simulink model "PneumaticsSystem"  (R2019b)
settings: configuration reference "ConfigSet_PneumaticsSystem_Reference" (kept outside this file)
PostLoadFcn:
  | set_up_test_model()
model workspace (MAT data in the model file):
  PAtm = 101300
  Prm_PneumaticsSystem : Simulink.Parameter (value not decoded)
  SampleTime = 0.01
symbols that are objects in the model workspace (value not decoded): Prm_PneumaticsSystem
undefined symbols (not defined in the file): AirSuspensionBogie1Deflated, AirSuspensionPressure, AirSuspensionPressureSwitch, AirSuspPressureDiff, AuxiliaryReservoirPressure, AuxiliaryReservoirPressureSwitch, BECU1BrakeNotApplied, BECU1BrakeNotReleased, BECU1CarLoadPressureLow, BECU1EmergencyBrakeFailure, BECU1LoadPressureLow, BECU1ServiceBrakeFailure, BECU2CarLoadPressureLow, BECU2EmergencyBrakeFailure, BECULowRPressure, Bogie, BrakeCylinderControlPressure, BrakeCylinderPressure, BrakeCylinderPressureGauge, BrakeCylinderPressureSwitch, BrakeReservoirPressure, BrakeReservoirPressureSwitch, HornHighPressureSwitch, HornLowPressureSwitch, MainReservoirPipePressure, MainReservoirPipePressureSwitch, MainReservoirPressure, MainReservoirPressureGauge, MainReservoirPressureSwitch, MaxAxles, MRPS_TractionCutout, ORDPressureSwitch, PantographCylinderPressure, ParkBrakePressure, ParkBrakePressureGauge, ParkBrakePressureSwitch, PS2, PS3, SandingSystemPressure, SandingSystemPressureSwitch, SRPressureGauge, VCBCylinderPressure, VCBPressureSwitch
libraries: PneumaticLib x56, simulink x50, LatchesLib x7, FiltersLib x4, TimersLib x3, MathOperationsLib x3, VectorOperationsLib x1, simulink_extras x1
(part 3 of 3)

== system PneumaticsSystem/PneumaticsPerVehicle/PneumaticsSystem/MainReservoirSystem/MainReservoirPipe/FlowCalc ==
  MRPSelf : Inport
  MRPUpPressure : Inport  Port=2
  MRPDownPressure : Inport  Port=3
  MRPUpConnection : Inport  Port=4
  MRPDownConnection : Inport  Port=5
  MRPToBRFlowRate : Inport  Port=6
  MRPToAirSuspFlowRate : Inport  Port=7
  MRPToAuxRFlowRate : Inport  Port=8
  MRPToMRFlowRate : Inport  Port=9
  Add : Sum  Inputs=------
  Logical Operator : Logic  Operator=NOT  AllPortsSameDT=off  OutDataTypeStr=boolean
  Logical Operator1 : Logic  Operator=NOT  AllPortsSameDT=off  OutDataTypeStr=boolean
  MRP to Downstream Connection : PneumaticLib/SS Two Way Valve  d=0.01475  p_deadband=200
      settings: SourceProductName=Pneumatic
  MRP to Upstream Connection : PneumaticLib/SS Two Way Valve  d=0.01475  p_deadband=200
      settings: SourceProductName=Pneumatic
  Terminator1 : Terminator
  Terminator2 : Terminator
  Flow : Outport  VectorParamsAs1DForOutWhenUnconnected=off
  wires:
  Add/1 -> Flow/1  "flowMRP"
  MRPDownPressure/1 -> MRP to Downstream Connection/2
  MRPDownConnection/1 -> Logical Operator1/1
  MRPUpConnection/1 -> Logical Operator/1
  MRPUpPressure/1 -> MRP to Upstream Connection/2
  MRP to Upstream Connection/2 -> Terminator2/1
  Logical Operator/1 -> MRP to Upstream Connection/3
  MRPSelf/1 -> MRP to Downstream Connection/1, MRP to Upstream Connection/1
  MRP to Upstream Connection/1 -> Add/1  "MRPUpPressureFlowRate"
  MRP to Downstream Connection/1 -> Add/2  "MRPDownPressureFlowRate"
  MRP to Downstream Connection/2 -> Terminator1/1
  Logical Operator1/1 -> MRP to Downstream Connection/3
  MRPToMRFlowRate/1 -> Add/4  "MRPToMRFlowRate"
  MRPToAirSuspFlowRate/1 -> Add/5  "MRPToAirSuspFlowRate"
  MRPToBRFlowRate/1 -> Add/3  "MRPToBRFlowRate"
  MRPToAuxRFlowRate/1 -> Add/6  "MRPToMRFlowRate"

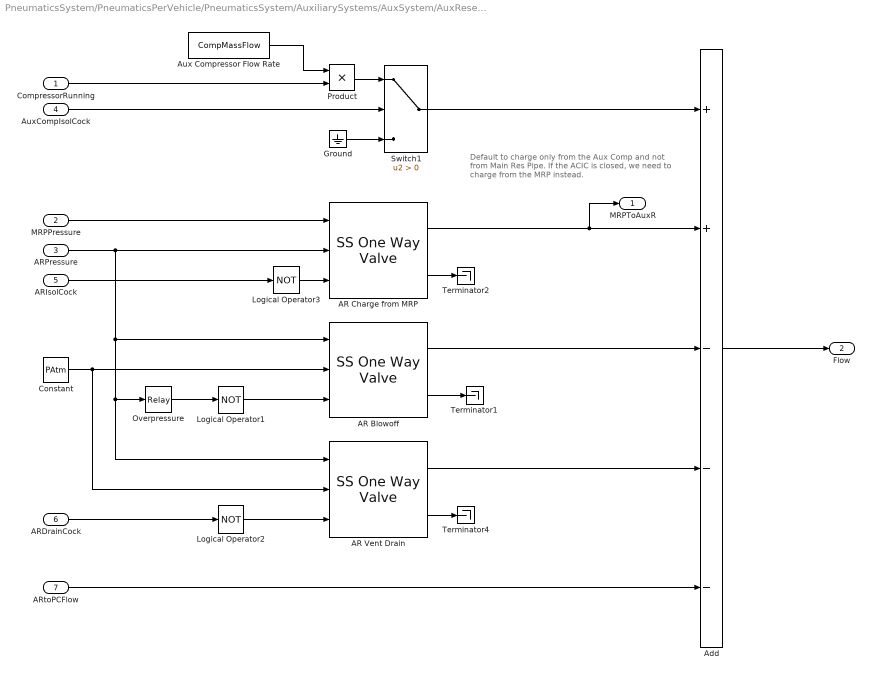
== system PneumaticsSystem/PneumaticsPerVehicle/PneumaticsSystem/AuxiliarySystems/AuxSystem/AuxReservoir/FlowCalc ==
  note: Default to charge only from the Aux Comp and not
      | from Main Res Pipe.
      | If the ACIC is closed, we need to charge from the
      | MRP instead.
  CompressorRunning : Inport
  MRPPressure : Inport  Port=2
  ARPressure : Inport  Port=3
  AuxCompIsolCock : Inport  Port=4
  ARIsolCock : Inport  Port=5
  ARDrainCock : Inport  Port=6
  ARtoPCFlow : Inport  Port=7
  AR Blowoff : PneumaticLib/SS One Way Valve  d=0.001  p_deadband=1000
      settings: SourceProductName=Train Library
  AR Charge from MRP : PneumaticLib/SS One Way Valve  d=0.0025  p_deadband=1000
      settings: SourceProductName=Train Library
  AR Vent Drain : PneumaticLib/SS One Way Valve  d=0.005  p_deadband=1000
      settings: SourceProductName=Train Library
  Add : Sum  Inputs=++---
  Aux Compressor Flow Rate : Constant  Value=CompMassFlow
  Constant : Constant  Value=PAtm
  Ground : Ground
  Logical Operator1 : Logic  Operator=NOT  AllPortsSameDT=off  OutDataTypeStr=boolean
  Logical Operator2 : Logic  Operator=NOT  AllPortsSameDT=off  OutDataTypeStr=boolean
  Logical Operator3 : Logic  Operator=NOT  AllPortsSameDT=off  OutDataTypeStr=boolean
  Overpressure : Relay  OnSwitchValue=BlowOffON + PAtm  OffSwitchValue=BlowOffOFF + PAtm
  Product : Product
  Switch1 : Switch  Criteria=u2 > Threshold
  Terminator1 : Terminator
  Terminator2 : Terminator
  Terminator4 : Terminator
  MRPToAuxR : Outport
  Flow : Outport  Port=2
  wires:
  Logical Operator2/1 -> AR Vent Drain/3
  AR Vent Drain/2 -> Terminator4/1
  Constant/1 -> AR Blowoff/2, AR Vent Drain/2
  AR Blowoff/2 -> Terminator1/1
  Add/1 -> Flow/1
  ARPressure/1 -> AR Vent Drain/1, Overpressure/1, AR Blowoff/1, AR Charge from MRP/2
  Overpressure/1 -> Logical Operator1/1
  Logical Operator1/1 -> AR Blowoff/3
  ARDrainCock/1 -> Logical Operator2/1
  MRPPressure/1 -> AR Charge from MRP/1
  ARtoPCFlow/1 -> Add/5
  AR Charge from MRP/2 -> Terminator2/1
  Product/1 -> Switch1/1
  AR Blowoff/1 -> Add/3
  AR Vent Drain/1 -> Add/4
  AuxCompIsolCock/1 -> Switch1/2
  AR Charge from MRP/1 -> MRPToAuxR/1, Add/2
  Aux Compressor Flow Rate/1 -> Product/1
  CompressorRunning/1 -> Product/2
  Ground/1 -> Switch1/3
  Switch1/1 -> Add/1
  ARIsolCock/1 -> Logical Operator3/1
  Logical Operator3/1 -> AR Charge from MRP/3

== system PneumaticsSystem/PneumaticsPerVehicle/PneumaticsSystem/AuxiliarySystems/AuxSystem/Pantograph/BellowCylinder ==
  InFlow : Inport
  Reset : Inport  Port=2
  AirBellowPressureSafegaurd : PneumaticLib/Limited Air Pressure Vessel  resetPrs=PAtm+ResetPressure
      settings: SourceProductName=Pneumatic
  Constant1 : Constant  Value=PAtm+MaxPressure
  Constant2 : Constant  Value=false  OutDataTypeStr=boolean
  Terminator1 : Terminator
  pAtm1 : Constant  Value=PAtm
  pAtm3 : Constant  Value=Volume
  BellowSafegaurdPressure : Outport
  wires:
  Constant1/1 -> AirBellowPressureSafegaurd/3
  AirBellowPressureSafegaurd/2 -> Terminator1/1
  pAtm1/1 -> AirBellowPressureSafegaurd/7, AirBellowPressureSafegaurd/4
  pAtm3/1 -> AirBellowPressureSafegaurd/2
  AirBellowPressureSafegaurd/1 -> BellowSafegaurdPressure/1  "BellowSafegaurdPressure"
  InFlow/1 -> AirBellowPressureSafegaurd/1
  Constant2/1 -> AirBellowPressureSafegaurd/5
  Reset/1 -> AirBellowPressureSafegaurd/6

== system PneumaticsSystem/PneumaticsPerVehicle/PneumaticsSystem/AuxiliarySystems/AuxSystem/Pantograph/FlowCalc ==
  note: There should probably be a regulator here for the supply pressures (from MRP and ARP)
  Fault : Inport
  ARPressure : Inport  Port=2
  PCPressure : Inport  Port=3
  PantoAirSupplyIsolCock : Inport  Port=4
  PantoControlValve : Inport  Port=5
  PantoEmerValve : Inport  Port=6
  AR Charge : PneumaticLib/SS One Way Valve  d=0.0025  p_deadband=1000
      settings: SourceProductName=Train Library
  Add : Sum  Inputs=+---
  Bus Selector3 : BusSelector  OutputSignals=PantographPipeLowPressure,ORDIntervention
  Constant : Constant  Value=PAtm
  Logical Operator : Logic  Operator=OR  Inputs=3  AllPortsSameDT=off  OutDataTypeStr=boolean
  Logical Operator1 : Logic  Operator=NOT  AllPortsSameDT=off  OutDataTypeStr=boolean
  Logical Operator5 : Logic  Operator=NAND  Inputs=3  AllPortsSameDT=off  OutDataTypeStr=boolean
  Logical Operator6 : Logic  Operator=NOT  AllPortsSameDT=off  OutDataTypeStr=boolean
  PC Vent Control : PneumaticLib/SS One Way Valve  d=0.0025  p_deadband=1000
      settings: SourceProductName=Train Library
  PC Vent Emer : PneumaticLib/SS One Way Valve  d=0.004  p_deadband=500
      settings: SourceProductName=Train Library
  PC Vent Isol : PneumaticLib/SS One Way Valve  d=0.004  p_deadband=500
      settings: SourceProductName=Train Library
  Product : Product
  Terminator{2..5} (4 alike) : Terminator
  Flow : Outport
  ARtoPCFlow : Outport  Port=2
  VentToBellow : Outport  Port=3
  wires:
  PC Vent Emer/2 -> Terminator3/1
  Logical Operator6/1 -> PC Vent Emer/3
  AR Charge/1 -> ARtoPCFlow/1, Add/1
  Logical Operator5/1 -> AR Charge/3
  PC Vent Control/1 -> Add/2
  AR Charge/2 -> Terminator2/1
  ARPressure/1 -> AR Charge/1
  PCPressure/1 -> AR Charge/2, PC Vent Control/1, PC Vent Isol/1, PC Vent Emer/1
  Add/1 -> Flow/1
  Constant/1 -> PC Vent Control/2, PC Vent Emer/2, PC Vent Isol/2
  PC Vent Control/2 -> Terminator4/1
  PantoControlValve/1 -> Logical Operator5/2, PC Vent Control/3
  PantoAirSupplyIsolCock/1 -> Logical Operator5/1, PC Vent Isol/3
  PantoEmerValve/1 -> Logical Operator/1
  PC Vent Emer/1 -> Product/1, Add/3
  PC Vent Isol/2 -> Terminator5/1
  PC Vent Isol/1 -> Add/4
  Fault/1 -> Bus Selector3/1
  Logical Operator/1 -> Logical Operator6/1
  Bus Selector3/1 -> Logical Operator/2  "<PantographPipeLowPressure>"
  Bus Selector3/2 -> Logical Operator1/1, Logical Operator/3, Product/2  "<ORDIntervention>"
  Logical Operator1/1 -> Logical Operator5/3
  Product/1 -> VentToBellow/1

== system PneumaticsSystem/PneumaticsPerVehicle/PneumaticsSystem/AuxiliarySystems/AuxSystem/Pantograph/PantoValves ==
  PantoRaiseValve : Inport
  PantoEmerVentValve : Inport  Port=2
  PantoPressureSwitch : Inport  Port=3
  Detect Change : simulink/Logic and Bit Operations/Detect Change  vinit=0  OutDataTypeStr=boolean
  Logical Operator : Logic  AllPortsSameDT=off  OutDataTypeStr=boolean
  S-R Flip-Flop : simulink_extras/Flip Flops/S-R Flip-Flop  initial_condition=0
  Terminator : Terminator
  PanControlValve : Outport
  PanEmergencyVentValve : Outport  Port=2
  wires:
  PantoRaiseValve/1 -> Detect Change/1, PanControlValve/1
  S-R Flip-Flop/1 -> PanEmergencyVentValve/1
  PantoPressureSwitch/1 -> Logical Operator/1
  PantoEmerVentValve/1 -> Logical Operator/2
  Logical Operator/1 -> S-R Flip-Flop/1
  Detect Change/1 -> S-R Flip-Flop/2
  S-R Flip-Flop/2 -> Terminator/1

== system PneumaticsSystem/PneumaticsPerVehicle/PneumaticsSystem/AuxiliarySystems/AuxSystem/Pantograph/StartupStateOverrideElectric ==
  note: Only at Initialisation
  PantoControlValve : Inport
  ARPressure : Inport  Port=2
  Constant1 : Constant  Value=true  OutDataTypeStr=boolean
  Ground : Ground
  Logical Operator33 : Logic  AllPortsSameDT=off  OutDataTypeStr=boolean
  NOT : Logic  Operator=NOT  AllPortsSameDT=off  OutDataTypeStr=boolean
  Switch : Switch  Criteria=u2 > Threshold
  Unit Delay1 : UnitDelay  SampleTime=-1  HasFrameUpgradeWarning=on
  Preset : Outport
  PresetVal : Outport  Port=2
  wires:
  Logical Operator33/1 -> Switch/2, Preset/1
  PantoControlValve/1 -> Logical Operator33/1
  Ground/1 -> Switch/3
  Switch/1 -> PresetVal/1
  ARPressure/1 -> Switch/1
  Unit Delay1/1 -> NOT/1
  NOT/1 -> Logical Operator33/2
  Constant1/1 -> Unit Delay1/1

== system PneumaticsSystem/PneumaticsPerVehicle/PneumaticsSystem/AuxiliarySystems/AuxSystem/VCB/Subsystem ==
  ARP : Inport
  VCBP : Inport  Port=2
  VCBCloseCmd : Inport  Port=3
  VCBIsolationCock : Inport  Port=4
  Logical Operator3 : Logic  Operator=NAND  AllPortsSameDT=off  OutDataTypeStr=boolean
  Sum : Sum  Inputs=+--
  Terminator : Terminator
  Terminator1 : Terminator
  Terminator2 : Terminator
  VCB Charge : PneumaticLib/SS One Way Valve  d=0.0025  p_deadband=1000
      settings: SourceProductName=Train Library
  VCB Isolate : PneumaticLib/SS One Way Valve  d=0.0025  p_deadband=1000
      settings: SourceProductName=Train Library
  VCB Vent : PneumaticLib/SS One Way Valve  d=0.0025  p_deadband=1000
      settings: SourceProductName=Train Library
  pAtm : Constant  Value=PAtm
  ARToVCB : Outport
  Flow : Outport  Port=2
  wires:
  VCB Charge/1 -> ARToVCB/1, Sum/1
  VCB Charge/2 -> Terminator/1
  VCBP/1 -> VCB Isolate/1, VCB Vent/1, VCB Charge/2
  ARP/1 -> VCB Charge/1
  Sum/1 -> Flow/1
  VCB Vent/1 -> Sum/2
  VCB Vent/2 -> Terminator1/1
  pAtm/1 -> VCB Isolate/2, VCB Vent/2
  VCB Isolate/2 -> Terminator2/1
  VCB Isolate/1 -> Sum/3
  VCBCloseCmd/1 -> Logical Operator3/1, VCB Vent/3
  Logical Operator3/1 -> VCB Charge/3
  VCBIsolationCock/1 -> Logical Operator3/2, VCB Isolate/3

== system PneumaticsSystem/PneumaticsPerVehicle/PneumaticsSystem/BogiePneumaticSystems/AirSuspensionSystem/AirSuspensionPerBogie/AirLevelingValve ==
  AirSuspensionPressure : Inport
  LoadPressureAbnormal : Inport  Port=2
  BogieSupportedMass : Inport  Port=3
  Abs : Abs
  Bias : Bias  Bias=PAtm
  Compare To Constant : simulink/Logic and Bit Operations/Compare To Constant  relop=>  const=2500  OutDataTypeStr=boolean
  Constant : Constant  Value=LoadCompensationMasses
  Constant1 : Constant  Value=LoadCompensationPressures
  Lookup Table Dynamic1 : simulink/Lookup Tables/Lookup Table Dynamic  LookUpMeth=Interpolation-Use End Values  OutDataType=fixdt('double')  OutScaling=[]  OutputDataTypeScalingMode=Specify via dialog  OutDataTypeStr=fixdt('double')  DoSatur=off
      settings: SourceProductName=Simulink
  NOT : Logic  Operator=NOT  AllPortsSameDT=off  OutDataTypeStr=boolean
  Product : Product  Inputs=3
  Sign : Signum
  Subtract : Sum  Inputs=+-
  limiter1 : Saturate  UpperLimit=MaxPressure + PAtm  LowerLimit=PAtm
  TargetPressure : Outport
  AirSuspensionValve : Outport  Port=2
  wires:
  AirSuspensionPressure/1 -> Subtract/2
  BogieSupportedMass/1 -> Lookup Table Dynamic1/1
  Product/1 -> AirSuspensionValve/1
  Constant/1 -> Lookup Table Dynamic1/2
  Constant1/1 -> Lookup Table Dynamic1/3
  Subtract/1 -> Abs/1, Sign/1
  Lookup Table Dynamic1/1 -> limiter1/1
  Abs/1 -> Compare To Constant/1
  limiter1/1 -> Bias/1
  Sign/1 -> Product/2
  Compare To Constant/1 -> Product/1
  Bias/1 -> TargetPressure/1, Subtract/1
  LoadPressureAbnormal/1 -> NOT/1
  NOT/1 -> Product/3

== system PneumaticsSystem/PneumaticsPerVehicle/PneumaticsSystem/BogiePneumaticSystems/AirSuspensionSystem/AirSuspensionPerBogie/FlowCalc ==
  AirSuspensionSupplyPressure : Inport
  AirSuspensionPressure : Inport  Port=2
  TargetPressure : Inport  Port=3
  AirSuspensionValve : Inport  Port=4
  AirSuspensionIsolCock : Inport  Port=5
  AirSuspensionDrainCock : Inport  Port=6
  AS Charge : PneumaticLib/SS One Way Valve Variable  p_deadband=1
      settings: SourceProductName=Train Library
  AS Vent : PneumaticLib/SS One Way Valve Variable  p_deadband=1
      settings: SourceProductName=Train Library
  AS Vent Drain : PneumaticLib/SS One Way Valve  d=0.015  p_deadband=1000
      settings: SourceProductName=Train Library
  AS Vent IC : PneumaticLib/SS One Way Valve  d=0.015  p_deadband=1000
      settings: SourceProductName=Train Library
  Add : Sum  Inputs=+---
  Charge Choke : PneumaticLib/Variable Orifice  FullDiam=0.005  DiffGain=0.0015
      settings: SourceProductName=Train Library
  Compare To Constant : simulink/Logic and Bit Operations/Compare To Constant  relop=~=  const=-1  OutDataTypeStr=boolean
  Compare To Constant1 : simulink/Logic and Bit Operations/Compare To Constant  relop=~=  const=1  OutDataTypeStr=boolean
  Constant : Constant  Value=PAtm
  Logical Operator2 : Logic  Operator=NOT  AllPortsSameDT=off  OutDataTypeStr=boolean
  Logical Operator4 : Logic  Operator=NOT  AllPortsSameDT=off  OutDataTypeStr=boolean
  Logical Operator5 : Logic  Operator=OR  AllPortsSameDT=off  OutDataTypeStr=boolean
  Release Choke : PneumaticLib/Variable Orifice  FullDiam=0.007  DiffGain=0.0015
      settings: SourceProductName=Train Library
  Terminator{,1,4..5} (4 alike) : Terminator
  ASRToAS : Outport
  Flow : Outport  Port=2
  wires:
  TargetPressure/1 -> Release Choke/2, Charge Choke/1
  AS Charge/1 -> ASRToAS/1, Add/1
  Add/1 -> Flow/1
  AS Charge/2 -> Terminator/1
  AS Vent/2 -> Terminator1/1
  AS Vent/1 -> Add/2
  AirSuspensionSupplyPressure/1 -> AS Charge/1
  Charge Choke/1 -> AS Charge/3
  Release Choke/1 -> AS Vent/3
  AirSuspensionDrainCock/1 -> Logical Operator2/1
  AS Vent IC/2 -> Terminator4/1
  AS Vent IC/1 -> Add/3
  AirSuspensionPressure/1 -> AS Charge/2, Charge Choke/2, AS Vent/1, AS Vent IC/1, AS Vent Drain/1, Release Choke/1
  Constant/1 -> AS Vent/2, AS Vent IC/2, AS Vent Drain/2
  AS Vent Drain/2 -> Terminator5/1
  AS Vent Drain/1 -> Add/4
  Logical Operator2/1 -> AS Vent Drain/3
  Compare To Constant/1 -> AS Vent/4
  Logical Operator5/1 -> AS Charge/4
  Logical Operator4/1 -> Logical Operator5/1
  AirSuspensionValve/1 -> Compare To Constant/1, Compare To Constant1/1
  Compare To Constant1/1 -> Logical Operator5/2
  AirSuspensionIsolCock/1 -> AS Vent IC/3, Logical Operator4/1

== system PneumaticsSystem/PneumaticsPerVehicle/PneumaticsSystem/BogiePneumaticSystems/AirSuspensionSystem/AirSuspensionPerBogie/Subsystem ==
  CarLoadPressureLow : Inport
  <BECU1LoadPressureLow> : Inport  Port=2
  <AirSuspensionBogie1Deflated> : Inport  Port=3
  Pressure : Inport  Port=4
  TargetPressure : Inport  Port=5
  Abs : Abs
  Constant : Constant  Value=0
  First Order Low Pass Filter : FiltersLib/First Order Low Pass Filter  FilterSpecificationSource=internal  FilterSpecificationType=Specify Time Constant  FilterSpecificationValue=0.1  SampleTime=-1
      settings: SourceProductName=Filters
  Gain : Gain  Gain=0.7
  Gain1 : Gain  Gain=0.5
  Gain2 : Gain  Gain=100
  SafeDivide : MathOperationsLib/SafeDivide
      settings: SourceProductName=Math Operations
  Subtract : Sum  Inputs=+-
  Switch : Switch  Criteria=u2 > Threshold
  Switch1 : Switch  Criteria=u2 > Threshold
  Switch2 : Switch  Criteria=u2 > Threshold
  PressureOut : Outport
  AirSuspPressure%Variation : Outport  Port=2
  wires:
  <AirSuspensionBogie1Deflated>/1 -> Switch2/2
  CarLoadPressureLow/1 -> Switch/2
  Switch2/1 -> First Order Low Pass Filter/1
  Gain/1 -> Switch/1
  Constant/1 -> Switch2/1
  Switch1/1 -> Switch2/3
  Switch/1 -> Switch1/3
  <BECU1LoadPressureLow>/1 -> Switch1/2
  Gain1/1 -> Switch1/1
  Pressure/1 -> Switch/3, Gain1/1, Gain/1
  Abs/1 -> AirSuspPressure%Variation/1
  First Order Low Pass Filter/1 -> Subtract/2, PressureOut/1
  Subtract/1 -> SafeDivide/1
  TargetPressure/1 -> SafeDivide/2, Subtract/1
  SafeDivide/1 -> Gain2/1
  Gain2/1 -> Abs/1

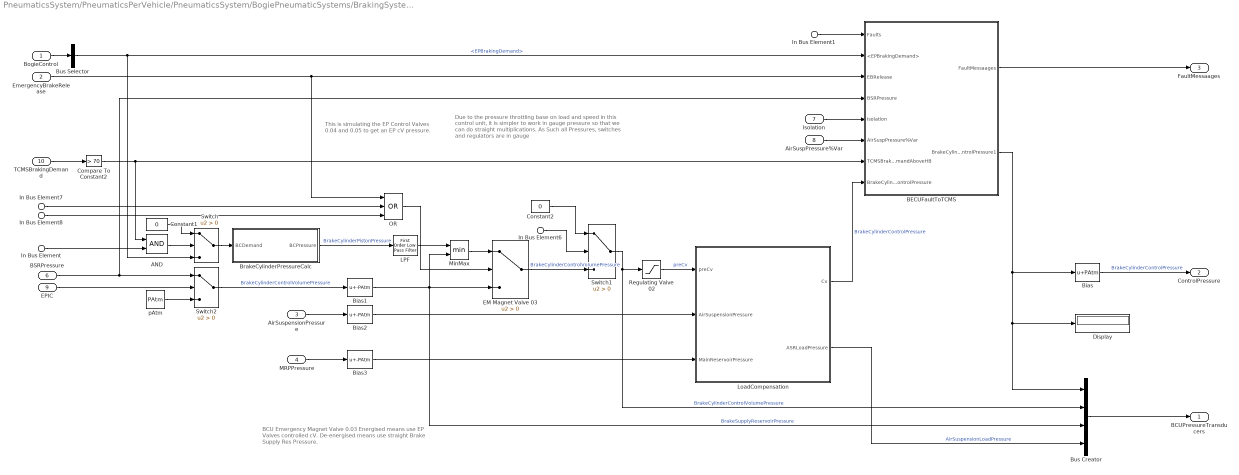
== system PneumaticsSystem/PneumaticsPerVehicle/PneumaticsSystem/BogiePneumaticSystems/BrakingSystem/BrakingSystemPerBogie/BrakeControlUnit ==
  note: Due to the pressure throttling base on load and speed
      | in this control unit, it is simpler to work in gauge pressure
      | so that we can do straight multiplications.
      |
      | As Such all Pressures, switches and regulators are in gauge
  note: BCU Emergency Magnet Valve 0.03
      | Energised means use EP Valves controlled cV.
      | De-energised means use straight Brake Supply Res Pressure.
  note: This is simulating the EP Control Valves
      | 0.04 and 0.05 to get an EP cV pressure.
  BogieControl : Inport
  EmergencyBrakeRelease : Inport  Port=2
  AirSuspensionPressure : Inport  Port=3
  MRPPressure : Inport  Port=4
  In Bus Element1 : Inport  Port=5  PortName=Faults
  In Bus Element : Inport  Port=5  PortName=Faults  Element=BECU1ServiceBrakeFailure
  In Bus Element7 : Inport  Port=5  PortName=Faults  Element=BECU1EmergencyBrakeFailure
  In Bus Element8 : Inport  Port=5  PortName=Faults  Element=BECU2EmergencyBrakeFailure
  In Bus Element6 : Inport  Port=5  PortName=Faults  Element=BECU1BrakeNotApplied
  BSRPressure : Inport  Port=6
  Isolation : Inport  Port=7
  AirSuspPressure%Var : Inport  Port=8
  EPIC : Inport  Port=9
  TCMSBrakingDemand : Inport  Port=10
  AND : Logic  AllPortsSameDT=off  OutDataTypeStr=boolean
  BECUFaultToTCMS : Subsystem
  Bias : Bias  Bias=PAtm
  Bias1 : Bias  Bias=-PAtm
  Bias2 : Bias  Bias=-PAtm
  Bias3 : Bias  Bias=-PAtm
  BrakeCylinderPressureCalc : Subsystem  mask{bcPreload=5000, noBrakeCyl=4, bcArea=0.024, brkBeamFactor=1, brkEfficiency=95, pAtm=PAtm}
      mask prompts: bcPreload "Brake cylinder preload (Pa)"; noBrakeCyl "Number of brake cylinders"; bcArea "Brake cylinder piston area (m^2)"; brkBeamFactor "Brake beam factor"; brkEfficiency "Brake efficiency (%)"; pAtm "Atmospheric pressure (Pa)"
  Bus Creator : BusCreator  Inputs=4  OutDataTypeStr=Bus: BD_PneumaticsSystem_Out_Vehicle_Transducers_Bogie  NonVirtualBus=on
      settings: InheritFromInputs=off
  Bus Selector : BusSelector  OutputSignals=EPBrakingDemand
  Compare To Constant2 : simulink/Logic and Bit Operations/Compare To Constant  relop=>  const=70  OutDataTypeStr=boolean
  Constant1 : Constant  Value=0
  Constant2 : Constant  Value=0
  Display : Display
  EM Magnet Valve 03 : Switch  Criteria=u2 > Threshold
  LPF : FiltersLib/First Order Low Pass Filter  FilterSpecificationSource=internal  FilterSpecificationType=Specify Time Constant  FilterSpecificationValue=0.1  SampleTime=-1
      settings: SourceProductName=Filters
  LoadCompensation : Subsystem
  MinMax : MinMax  Inputs=2
  OR : Logic  Operator=OR  Inputs=3  AllPortsSameDT=off  OutDataTypeStr=boolean
  Regulating Valve 02 : Saturate  UpperLimit=MaxControlPressure  LowerLimit=0
  Switch : Switch  Criteria=u2 > Threshold
  Switch1 : Switch  Criteria=u2 > Threshold
  Switch2 : Switch  Criteria=u2 > Threshold
  pAtm : Constant  Value=PAtm
  BCUPressureTransducers : Outport
  ControlPressure : Outport  Port=2
  FaultMessaages : Outport  Port=3
  wires:
  MinMax/1 -> EM Magnet Valve 03/1
  LPF/1 -> MinMax/1
  MRPPressure/1 -> Bias3/1
  Switch1/1 -> Bus Creator/2, Regulating Valve 02/1  "BrakeCylinderControlVolumePressure"
  EmergencyBrakeRelease/1 -> OR/1, BECUFaultToTCMS/3(EBRelease)
  Bias3/1 -> LoadCompensation/3(MainReservoirPressure)
  AirSuspensionPressure/1 -> Bias2/1
  Bias2/1 -> LoadCompensation/2(AirSuspensionPressure)
  LoadCompensation/2(ASRLoadPressure) -> Bus Creator/4  "AirSuspensionLoadPressure"
  Regulating Valve 02/1 -> LoadCompensation/1(preCv)  "preCv"
  BSRPressure/1 -> BECUFaultToTCMS/4(BSRPressure), Switch2/1
  Bias1/1 -> Bus Creator/3, EM Magnet Valve 03/3, MinMax/2  "BrakeSupplyReservoirPressure"
  Bus Creator/1 -> BCUPressureTransducers/1
  Bias/1 -> ControlPressure/1  "BrakeCylinderControlPressure"
  BogieControl/1 -> Bus Selector/1
  Bus Selector/1 -> BECUFaultToTCMS/2(<EPBrakingDemand>), Switch/3  "<EPBrakingDemand>"
  BrakeCylinderPressureCalc/1(BCPressure) -> LPF/1  "BrakeCylinderPistonPressure"
  Constant1/1 -> Switch/1
  Switch/1 -> BrakeCylinderPressureCalc/1(BCDemand)
  In Bus Element6/1 -> Switch1/2
  In Bus Element/1 -> AND/2
  BECUFaultToTCMS/2(BrakeCylinderControlPressure1) -> Bus Creator/1, Display/1, Bias/1
  LoadCompensation/1(Cv) -> BECUFaultToTCMS/8(BrakeCylinderControlPressure)  "BrakeCylinderControlPressure"
  BECUFaultToTCMS/1(FaultMessaages) -> FaultMessaages/1
  Constant2/1 -> Switch1/1
  EM Magnet Valve 03/1 -> Switch1/3  "BrakeCylinderControlVolumePressure"
  Isolation/1 -> BECUFaultToTCMS/5(Isolation)
  In Bus Element7/1 -> OR/2
  In Bus Element8/1 -> OR/3
  OR/1 -> EM Magnet Valve 03/2
  In Bus Element1/1 -> BECUFaultToTCMS/1(Faults)
  AirSuspPressure%Var/1 -> BECUFaultToTCMS/6(AirSuspPressure%Var)
  Switch2/1 -> Bias1/1  "BrakeCylinderControlVolumePressure"
  EPIC/1 -> Switch2/2
  pAtm/1 -> Switch2/3
  TCMSBrakingDemand/1 -> Compare To Constant2/1
  AND/1 -> Switch/2
  Compare To Constant2/1 -> AND/1, BECUFaultToTCMS/7(TCMSBrakingDemandAboveHB)

== system PneumaticsSystem/PneumaticsPerVehicle/PneumaticsSystem/BogiePneumaticSystems/BrakingSystem/BrakingSystemPerBogie/BrakeCylinderSupplyLine ==
  note: The Bogie BC Pressure Gauge is tapped off the Brake Cylinder supply line after the Brake Cylidner Isolation Cock.
      | We are not specifically modelling this portion of pipe so we will do a local calculation.
      | This will take the average of the Control pressure or Atmospheric depending on the BC Isolation Cock,
      | and each of the Brake Cylinder pressures.
  BCPressures : Inport
  ControlPressure : Inport  Port=2
  BCIsolCock : Inport  Port=3
  BrakeCylindersPerAxle : Inport  Port=4
  Atmospheric : Constant  Value=PAtm
  B27/28-B07 : PneumaticLib/Pressure Switch  OnSwitchValue=PressureSwitchON  OffSwitchValue=PressureSwitchOFF  OnOutputValue=1  OffOutputValue=0  InitOn=on
      settings: SourceProductName=Train Library
  Bias : Bias  Bias=-PAtm
  HasBC : simulink/Logic and Bit Operations/Compare To Zero  relop=>  OutDataTypeStr=uint8
  LPF : FiltersLib/First Order Low Pass Filter  FilterSpecificationSource=internal  FilterSpecificationType=Specify Time Constant  FilterSpecificationValue=0.01  SampleTime=-1
      settings: SourceProductName=Filters
  Mean of Elements : MathOperationsLib/Mean of Elements
      settings: SourceProductName=Math Operations
  SafeDivide : MathOperationsLib/SafeDivide
      settings: SourceProductName=Math Operations
  Sum of Elements : Sum  Inputs=+
  Sum of Elements1 : Sum  Inputs=+
  Switch : Switch  Criteria=u2 > Threshold
  Switch1 : Switch  Criteria=u2 > Threshold
  Vector Concatenate : Concatenate
  Vector Concatenate1 : Concatenate
  BCPressureSwitch : Outport
  BCPressureGauge : Outport  Port=2
  BCSupplyLinePressure : Outport  Port=3
  wires:
  ControlPressure/1 -> Switch/1
  Vector Concatenate/1 -> Switch1/1
  Mean of Elements/1 -> LPF/1
  SafeDivide/1 -> Vector Concatenate/2
  BCIsolCock/1 -> Switch/2
  Atmospheric/1 -> Switch/3
  Switch/1 -> Vector Concatenate1/2, Vector Concatenate1/1, Vector Concatenate/1
  LPF/1 -> Bias/1, BCSupplyLinePressure/1
  Bias/1 -> B27/28-B07/1, BCPressureGauge/1  "BrakeCylinderPressureGauge"
  B27/28-B07/1 -> BCPressureSwitch/1  "BrakeCylinderPressureSwitch"
  Sum of Elements/1 -> SafeDivide/1
  BCPressures/1 -> Sum of Elements/1
  Sum of Elements1/1 -> SafeDivide/2, Switch1/2
  BrakeCylindersPerAxle/1 -> HasBC/1
  HasBC/1 -> Sum of Elements1/1
  Vector Concatenate1/1 -> Switch1/3
  Switch1/1 -> Mean of Elements/1

== system PneumaticsSystem/PneumaticsPerVehicle/PneumaticsSystem/BogiePneumaticSystems/BrakingSystem/BrakingSystemPerBogie/BrakeCylinderSystemPerAxle ==
  ControlPressure : Inport
  BSRPressure : Inport  Port=2
  Reset : Inport  Port=3
  BCIsolCock : Inport  Port=4
  BrakeCylindersPerAxle : Inport  Port=5  Partition=on  PartitionDimension=1  PartitionWidth=1  PartitionOffset=0
  AxleBrakeCylinder : Subsystem
  Compare To Zero : simulink/Logic and Bit Operations/Compare To Zero  relop=>  OutDataTypeStr=boolean
  For Each : ForEach  DisableCoverage=on
  BSRtoBCFlow : Outport  ConcatenationDimension=1
  BrakeCylinderPressure : Outport  Port=2  ConcatenationDimension=1
  wires:
  BSRPressure/1 -> AxleBrakeCylinder/1(BSRPressure)
  ControlPressure/1 -> AxleBrakeCylinder/2(ControlPressure)
  Reset/1 -> AxleBrakeCylinder/3(Reset)
  AxleBrakeCylinder/1(BCPressure) -> BrakeCylinderPressure/1  "BrakeCylinderPressure"
  BCIsolCock/1 -> AxleBrakeCylinder/4(BCIsolCock)
  AxleBrakeCylinder/2(BSRtoBCFlow) -> BSRtoBCFlow/1
  BrakeCylindersPerAxle/1 -> Compare To Zero/1
  Compare To Zero/1 -> AxleBrakeCylinder/Enable

== system PneumaticsSystem/PneumaticsPerVehicle/PneumaticsSystem/BogiePneumaticSystems/BrakingSystem/BrakingSystemPerBogie/ParkBrakes ==
  note: Parking Force is applied when the pressure in the supply line is decreased below the Switch ON point.
      | Park Brake Apply Valve allows to apply parking brakes by venting the Park Brake Supply Line to atmosphere.
      | Park Brakes will only apply if Brake Cylinder are not already applying.
      | If the Park Brake Supply Line is isolated, it vents to atmosphere and therefore applies the Park Brakes.
      | In that state, to release the Park Brakes, operate the Manual Release.
      | To re-engage Park Brakes as normal, un-isolate the Park Brake Isolation Cock.
  BCSupplyLinePressure : Inport
  MRPPressure : Inport  Port=2
  PBApplyCmd : Inport  Port=3
  PBReleaseCmd : Inport  Port=4
  PBIsolCock : Inport  Port=5
  PBManualRelease : Inport  Port=6
  AND : Logic  AllPortsSameDT=off  OutDataTypeStr=boolean
  B27-B14 : PneumaticLib/Pressure Switch  OnSwitchValue=PressureSwitchON  OffSwitchValue=PressureSwitchOFF  OnOutputValue=0  OffOutputValue=1  InitOn=on
      settings: SourceProductName=Train Library
  Bias : Bias  Bias=-PAtm
  Bias1 : Bias  Bias=-PAtm
  Constant : Constant  Value=PAtm
  Constant1 : Constant  Value=PAtm
  DoubleCheckValve : MinMax  Function=max  Inputs=2
  LPF : FiltersLib/First Order Low Pass Filter  FilterSpecificationSource=internal  FilterSpecificationType=Specify Time Constant  FilterSpecificationValue=0.01  SampleTime=-1
      settings: SourceProductName=Filters
  MagnetValve_B20 : LatchesLib/SR Latch - Reset Priority  initial_condition=0
      settings: SourceProductName=Latches
  Max : MinMax  Function=max
  NOT : Logic  Operator=NOT  AllPortsSameDT=off  OutDataTypeStr=boolean
  PBPressures : Constant  Value=ParkingPressures
  Switch1 : Switch  Criteria=u2 > Threshold
  Switch2 : Switch  Criteria=u2 > Threshold
  Switch3 : Switch  Criteria=u2 > Threshold
  ParkBrakePressureGauge : Outport
  ParkBrakePressure : Outport  Port=2
  ParkBrakePressureSwitch : Outport  Port=3
  wires:
  DoubleCheckValve/1 -> Bias1/1, Switch3/1
  BCSupplyLinePressure/1 -> DoubleCheckValve/2
  MRPPressure/1 -> Switch1/3
  PBIsolCock/1 -> Switch3/2, NOT/1
  Constant/1 -> Switch3/3
  Switch3/1 -> Switch2/3
  LPF/1 -> ParkBrakePressure/1, Bias/1  "ParkBrakePressure"
  PBPressures/1 -> Max/1
  Bias/1 -> ParkBrakePressureGauge/1  "ParkBrakePressureGauge"
  B27-B14/1 -> ParkBrakePressureSwitch/1  "ParkBrakePressureSwitch"
  Constant1/1 -> Switch1/1
  MagnetValve_B20/1 -> Switch1/2
  Switch1/1 -> DoubleCheckValve/1  "ParkBrakeSupplyLine"
  NOT/1 -> AND/1
  AND/1 -> Switch2/2
  Max/1 -> Switch2/1
  Switch2/1 -> LPF/1
  PBApplyCmd/1 -> MagnetValve_B20/1
  PBReleaseCmd/1 -> MagnetValve_B20/2
  PBManualRelease/1 -> AND/2
  Bias1/1 -> B27-B14/1  "ParkBrakePressureGauge"

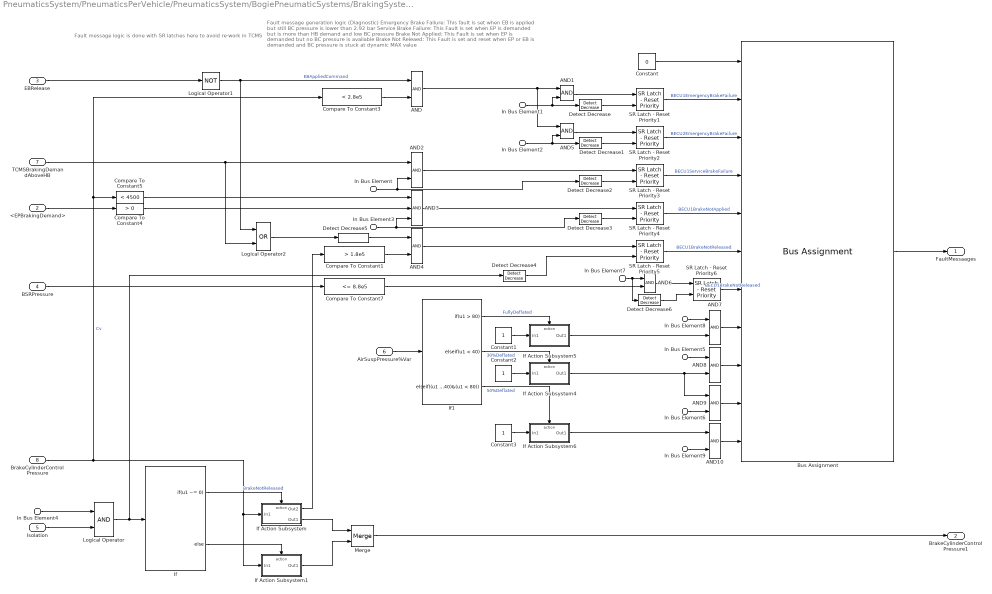
== system PneumaticsSystem/PneumaticsPerVehicle/PneumaticsSystem/BogiePneumaticSystems/BrakingSystem/BrakingSystemPerBogie/BrakeControlUnit/BECUFaultToTCMS ==
  note: Fault message generation logic (Diagnostic)
      | Emergency Brake Failure: This fault is set when EB is applied but still BC pressure is lower than 2.92 bar
      | Service Brake Failure: This Fault is set when EP is demanded but is more than HB demand and low BC pressure
      | Brake Not Applied: This Fault is set when EP is demanded but no BC pressure is available
      | Brake Not Releaed: This Fault is set and reset when EP or EB is demanded and BC pressure is stuck at dynamic MAX value
  note: Fault message logic is done with SR latches here to avoid re-work in TCMS
  In Bus Element5 : Inport  PortName=Faults  Element=BECU1CarLoadPressureLow
  In Bus Element6 : Inport  PortName=Faults  Element=BECU2CarLoadPressureLow
  In Bus Element7 : Inport  PortName=Faults  Element=BECULowRPressure
  In Bus Element3 : Inport  PortName=Faults  Element=BECU1BrakeNotApplied
  In Bus Element : Inport  PortName=Faults  Element=BECU1ServiceBrakeFailure
  In Bus Element2 : Inport  PortName=Faults  Element=BECU2EmergencyBrakeFailure
  In Bus Element1 : Inport  PortName=Faults  Element=BECU1EmergencyBrakeFailure
  In Bus Element4 : Inport  PortName=Faults  Element=BECU1BrakeNotReleased
  In Bus Element8 : Inport  PortName=Faults  Element=AirSuspensionBogie1Deflated
  In Bus Element9 : Inport  PortName=Faults  Element=BECU1LoadPressureLow
  <EPBrakingDemand> : Inport  Port=2
  EBRelease : Inport  Port=3
  BSRPressure : Inport  Port=4
  Isolation : Inport  Port=5
  AirSuspPressure%Var : Inport  Port=6
  TCMSBrakingDemandAboveHB : Inport  Port=7
  BrakeCylinderControlPressure : Inport  Port=8
  AND{,1..2,4..10} (10 alike) : Logic  AllPortsSameDT=off  OutDataTypeStr=boolean
  AND3 : Logic  Inputs=3  AllPortsSameDT=off  OutDataTypeStr=boolean
  Bus Assignment : BusAssignment  AssignedSignals=BECU1EmergencyBrakeFailure,BECU2EmergencyBrakeFailure,BECU1ServiceBrakeFailure,BECU1BrakeNotApplied,BECU1BrakeNotReleased,BECULowRPressure,AirSuspensionBogie1Deflated,BECU1CarLoadPressureLow,BECU2CarLoadPressureLow,BECU1LoadPressureLow
  Compare To Constant1 : simulink/Logic and Bit Operations/Compare To Constant  relop=>  const=1.8e5  OutDataTypeStr=boolean
  Compare To Constant3 : simulink/Logic and Bit Operations/Compare To Constant  relop=<  const=2.8e5  OutDataTypeStr=boolean
  Compare To Constant4 : simulink/Logic and Bit Operations/Compare To Constant  relop=>  const=0  OutDataTypeStr=boolean
  Compare To Constant5 : simulink/Logic and Bit Operations/Compare To Constant  relop=<  const=4500  OutDataTypeStr=boolean
  Compare To Constant7 : simulink/Logic and Bit Operations/Compare To Constant  relop=<=  const=8.8e5  OutDataTypeStr=boolean
  Constant : Constant  Value=0  OutDataTypeStr=Bus: BD_PneumaticsSystem_Out_Vehicle_TCMS_Bogie
  Constant1 : Constant
  Constant2 : Constant
  Constant3 : Constant
  Detect Decrease{,1..6} (7 alike) : simulink/Logic and Bit Operations/Detect Decrease  vinit=0.0  OutDataTypeStr=boolean
  If : If  IfExpression=u1 ~= 0
  If Action Subsystem : Subsystem  TreatAsAtomicUnit=on
  If Action Subsystem1 : Subsystem  TreatAsAtomicUnit=on
  If Action Subsystem4 : Subsystem  TreatAsAtomicUnit=on
  If Action Subsystem5 : Subsystem  TreatAsAtomicUnit=on
  If Action Subsystem6 : Subsystem  TreatAsAtomicUnit=on
  If1 : If  IfExpression=u1 > 80  ElseIfExpressions=u1 < 40, (u1 > 40)&(u1 < 80)  ShowElse=off
  Logical Operator : Logic  AllPortsSameDT=off  OutDataTypeStr=boolean
  Logical Operator1 : Logic  Operator=NOT  AllPortsSameDT=off  OutDataTypeStr=boolean
  Logical Operator2 : Logic  Operator=OR  AllPortsSameDT=off  OutDataTypeStr=boolean
  Merge : Merge
  SR Latch - Reset Priority{1..6} (6 alike) : LatchesLib/SR Latch - Reset Priority  initial_condition=0
      settings: SourceProductName=Latches
  FaultMessaages : Outport
  BrakeCylinderControlPressure1 : Outport  Port=2
  wires:
  Bus Assignment/1 -> FaultMessaages/1
  In Bus Element1/1 -> AND1/2, Detect Decrease/1
  SR Latch - Reset Priority1/1 -> Bus Assignment/2  "BECU1EmergencyBrakeFailure"
  In Bus Element4/1 -> Logical Operator/1
  SR Latch - Reset Priority4/1 -> Bus Assignment/5  "BECU1BrakeNotApplied"
  SR Latch - Reset Priority2/1 -> Bus Assignment/3  "BECU2EmergencyBrakeFailure"
  SR Latch - Reset Priority5/1 -> Bus Assignment/6  "BECU1BrakeNotReleased"
  SR Latch - Reset Priority3/1 -> Bus Assignment/4  "BECU1ServiceBrakeFailure"
  In Bus Element3/1 -> AND3/3, Detect Decrease3/1
  In Bus Element/1 -> AND2/2, Detect Decrease2/1
  Compare To Constant4/1 -> AND3/2
  BrakeCylinderControlPressure/1 -> If Action Subsystem1/1(In1), If Action Subsystem/1(In1), Compare To Constant5/1, Compare To Constant3/1  "Cv"
  <EPBrakingDemand>/1 -> Compare To Constant4/1
  Constant/1 -> Bus Assignment/1
  Isolation/1 -> Logical Operator/2
  AND/1 -> AND1/1, AND5/1
  AND2/1 -> SR Latch - Reset Priority3/1
  AND3/1 -> SR Latch - Reset Priority4/1
  AND4/1 -> SR Latch - Reset Priority5/1
  In Bus Element2/1 -> AND5/2, Detect Decrease1/1
  Logical Operator/1 -> Detect Decrease4/1, If/1
  EBRelease/1 -> Logical Operator1/1
  Logical Operator1/1 -> Logical Operator2/1, AND/1  "EBAppliedCommand"
  Detect Decrease/1 -> SR Latch - Reset Priority1/2
  Detect Decrease1/1 -> SR Latch - Reset Priority2/2
  AND5/1 -> SR Latch - Reset Priority2/1
  AND1/1 -> SR Latch - Reset Priority1/1
  Detect Decrease2/1 -> SR Latch - Reset Priority3/2
  Detect Decrease3/1 -> SR Latch - Reset Priority4/2
  Compare To Constant1/1 -> AND4/2
  Logical Operator2/1 -> Detect Decrease5/1
  Detect Decrease4/1 -> SR Latch - Reset Priority5/2
  Compare To Constant3/1 -> AND/2
  Detect Decrease5/1 -> AND4/1
  If/1 -> If Action Subsystem/Action  "BrakeNotReleased"
  If/2 -> If Action Subsystem1/Action
  Merge/1 -> BrakeCylinderControlPressure1/1
  If Action Subsystem1/1(Out1) -> Merge/2
  If Action Subsystem/2(Out1) -> Merge/1
  If Action Subsystem/1(Out2) -> Compare To Constant1/1
  Compare To Constant5/1 -> AND3/1
  AND8/1 -> Bus Assignment/9
  In Bus Element7/1 -> Detect Decrease6/1, AND6/1
  AND7/1 -> Bus Assignment/8
  AND6/1 -> SR Latch - Reset Priority6/1
  AirSuspPressure%Var/1 -> If1/1
  If1/3 -> If Action Subsystem6/Action  "50%Deflated"
  If1/1 -> If Action Subsystem5/Action  "FullyDeflated"
  If1/2 -> If Action Subsystem4/Action  "30%Deflated"
  Constant1/1 -> If Action Subsystem5/1(In1)
  Constant2/1 -> If Action Subsystem4/1(In1)
  Constant3/1 -> If Action Subsystem6/1(In1)
  AND10/1 -> Bus Assignment/11
  AND9/1 -> Bus Assignment/10
  If Action Subsystem5/1(Out1) -> AND7/2
  If Action Subsystem4/1(Out1) -> AND9/1, AND8/2
  If Action Subsystem6/1(Out1) -> AND10/1
  In Bus Element5/1 -> AND8/1
  In Bus Element6/1 -> AND9/2
  In Bus Element8/1 -> AND7/1
  In Bus Element9/1 -> AND10/2
  BSRPressure/1 -> Compare To Constant7/1
  Compare To Constant7/1 -> AND6/2
  TCMSBrakingDemandAboveHB/1 -> Logical Operator2/2, AND2/1
  SR Latch - Reset Priority6/1 -> Bus Assignment/7  "BECU1BrakeNotReleased"
  Detect Decrease6/1 -> SR Latch - Reset Priority6/2

== system PneumaticsSystem/PneumaticsPerVehicle/PneumaticsSystem/BogiePneumaticSystems/BrakingSystem/BrakingSystemPerBogie/BrakeControlUnit/BrakeCylinderPressureCalc ==
  note: Brake Cylinder Pressure
      | This block calculates the total braking pressure from the demand force input.
      | This back calculates the pressure, from the block used in braking system to convert pressure to force.
      | Braking force = (Cyl pressure - Patm - Preload)*CylArea*NoCyl*BeamFactor*(BrkEfficiency/100)
      | Cyl pressure = (Braking force/(CylArea*NoCyl*BeamFactor*(BrkEfficiency/100))) + Preload
  BCDemand : Inport
  Constant : Constant  Value=noBrakeCyl
  Constant1 : Constant  Value=bcArea
  Constant2 : Constant  Value=brkBeamFactor
  Constant3 : Constant  Value=brkEfficiency
  Constant4 : Constant  Value=100
  Constant5 : Constant  Value=bcPreload
  Product{1..5} (5 alike) : Product  Inputs=*/
  Sum : Sum
  BCPressure : Outport  VectorParamsAs1DForOutWhenUnconnected=off
  wires:
  Constant5/1 -> Sum/2
  Sum/1 -> BCPressure/1
  Product1/1 -> Product2/1
  Constant2/1 -> Product2/2
  Constant/1 -> Product5/2
  Product5/1 -> Product1/1
  Constant1/1 -> Product1/2
  Product2/1 -> Product3/1
  Constant3/1 -> Product4/1
  Product4/1 -> Product3/2
  BCDemand/1 -> Product5/1
  Constant4/1 -> Product4/2
  Product3/1 -> Sum/1

== system PneumaticsSystem/PneumaticsPerVehicle/PneumaticsSystem/BogiePneumaticSystems/BrakingSystem/BrakingSystemPerBogie/BrakeControlUnit/LoadCompensation ==
  note: The Load compensation valve takes Air Suspension Pressure
      | and reduces brake application pressure for lower loading.
      |
      | This could either be done as a proportion of the input pressure.
      | P_out = k * P_in
      |
      | or as a dynamic limiter
      | P_out = min(P_in, k * P_max)
      |
      | The first appiles load compensation to all input presusres (entire
      | service brakig and EB range). The second only applies to max input
      | pressure (EB only).
      |
      | For IEP, it seems service braking is load compensated in the demand
      | (such that ED braking is also load compnesated) And the Pneumatic
      | load compensation is for EB only.
  note: As load increases, Air Suspension pressure will increase,
      | which will in turn increase the Control Volume pressure
      | up to the maximum at crush load.
      |
      | If air pressure drops due to a leak, Control Volume pressure
      | will decrease until it hits the mimum at tare load.
      | It will continue using this minumum until the pressure drops
      | below 1 bar. At this point, regulated Main Res pressure of 6 bar will
      | be delivered to the Load Compensation relay valve, which increases
      | the Control Volume pressure back up to Maximum.
  note: The air suspension pressure may be a pressure from each bogie,
      | or two pressures from one bogie.
      | If both from one bogie and we are only modelling one air bag
      | per bogie, the width of the signal will be 1.
  preCv : Inport
  AirSuspensionPressure : Inport  Port=2
  MainReservoirPressure : Inport  Port=3
  Constant : Constant  Value=LoadCompensationGains
  Constant1 : Constant  Value=LoadCompensationPressures
  CrushRevertingPistonValve 02 : Switch  Threshold=PAtm
  Divide : Product  Inputs=*/
  Gain : Gain  Gain=MaxControlPressure
  Ground : Ground
  Ground1 : Ground
  LoadCompensatedEB : simulink/Discontinuities/Saturation Dynamic  OutMin=[]  OutMax=[]  OutDataTypeStr=Inherit: Same as second input  OutDataType=fixdt(1, 16)  OutScaling=2^-10  DoSatur=off
  Lookup Table Dynamic1 : simulink/Lookup Tables/Lookup Table Dynamic  LookUpMeth=Interpolation-Use End Values  OutDataType=fixdt('double')  OutScaling=[]  OutputDataTypeScalingMode=Specify via dialog  OutDataTypeStr=fixdt('double')  DoSatur=off
      settings: SourceProductName=Simulink
  Max : MinMax  Function=max
  Proportion : Saturate  UpperLimit=1  LowerLimit=0
  Regulating Valve : simulink/Discontinuities/Saturation Dynamic  OutMin=[]  OutMax=[]  OutDataTypeStr=Inherit: Same as second input  OutDataType=fixdt(1, 16)  OutScaling=2^-10  DoSatur=off
  Sum of Elements : Sum  Inputs=+
  Width : Width
  Cv : Outport
  ASRLoadPressure : Outport  Port=2
  wires:
  Lookup Table Dynamic1/1 -> Proportion/1
  Regulating Valve/1 -> CrushRevertingPistonValve 02/3
  CrushRevertingPistonValve 02/1 -> ASRLoadPressure/1, Lookup Table Dynamic1/1  "AirSuspensionLoadPressure"
  Sum of Elements/1 -> Divide/1
  Width/1 -> Divide/2
  Divide/1 -> CrushRevertingPistonValve 02/1, CrushRevertingPistonValve 02/2
  Proportion/1 -> Gain/1
  preCv/1 -> LoadCompensatedEB/2
  LoadCompensatedEB/1 -> Cv/1
  MainReservoirPressure/1 -> Regulating Valve/2
  AirSuspensionPressure/1 -> Width/1, Sum of Elements/1
  Constant1/1 -> Max/1, Lookup Table Dynamic1/2
  Constant/1 -> Lookup Table Dynamic1/3
  Gain/1 -> LoadCompensatedEB/1
  Ground/1 -> LoadCompensatedEB/3
  Max/1 -> Regulating Valve/1
  Ground1/1 -> Regulating Valve/3

== system PneumaticsSystem/PneumaticsPerVehicle/PneumaticsSystem/BogiePneumaticSystems/BrakingSystem/BrakingSystemPerBogie/BrakeCylinderSystemPerAxle/AxleBrakeCylinder ==
  BSRPressure : Inport
  ControlPressure : Inport  Port=2
  Reset : Inport  Port=3
  BCIsolCock : Inport  Port=4
  Enable : EnablePort
  Bias : Bias  Bias=-PAtm
  BrakeCylinder : PneumaticLib/Limited Air Pressure Vessel  resetPrs=PAtm + ResetPressure
      settings: SourceProductName=Pneumatic
  Constant : Constant  Value=PAtm + MaxPressure
  Constant1 : Constant  Value=true  OutDataTypeStr=boolean
  Display : Display
  FlowCalc : Subsystem
  NOT : Logic  Operator=NOT  AllPortsSameDT=off  OutDataTypeStr=boolean
  Terminator : Terminator
  Unit Delay : UnitDelay  SampleTime=-1  HasFrameUpgradeWarning=on
  Unit Delay1 : UnitDelay  SampleTime=-1  HasFrameUpgradeWarning=on
  pAtm : Constant  Value=PAtm
  pAtm2 : Constant  Value=Volume
  BCPressure : Outport
  BSRtoBCFlow : Outport  Port=2
  wires:
  pAtm2/1 -> BrakeCylinder/2
  ControlPressure/1 -> BrakeCylinder/7, FlowCalc/2(ControlPressure)
  pAtm/1 -> BrakeCylinder/4
  Reset/1 -> BrakeCylinder/5
  Unit Delay/1 -> FlowCalc/3(BCPressure)
  BSRPressure/1 -> FlowCalc/1(BSRPressure)
  Constant/1 -> BrakeCylinder/3
  BrakeCylinder/1 -> Unit Delay/1, Bias/1, BCPressure/1
  FlowCalc/1(Flow) -> BrakeCylinder/1
  Bias/1 -> Display/1
  BrakeCylinder/2 -> Terminator/1
  BCIsolCock/1 -> FlowCalc/4(BCIsolCock)
  FlowCalc/2(BSRtoBCFlow) -> BSRtoBCFlow/1
  Unit Delay1/1 -> NOT/1
  NOT/1 -> BrakeCylinder/6
  Constant1/1 -> Unit Delay1/1

== system PneumaticsSystem/PneumaticsPerVehicle/PneumaticsSystem/BogiePneumaticSystems/BrakingSystem/BrakingSystemPerBogie/BrakeControlUnit/BECUFaultToTCMS/If Action Subsystem ==
  In1 : Inport
  Action Port : ActionPort  ActionPortLabel=if(u1 ~= 0)
  Constant3 : Constant  Value=0
  Constant4 : Constant  Value=1e6
  Rate Limiter Dynamic2 : simulink/Discontinuities/Rate Limiter Dynamic
      settings: SourceProductName=Simulink
  Out2 : Outport  OutputWhenDisabled=reset  InitialOutput=0
  Out1 : Outport  Port=2
  wires:
  Constant3/1 -> Rate Limiter Dynamic2/3
  Constant4/1 -> Rate Limiter Dynamic2/1
  In1/1 -> Rate Limiter Dynamic2/2
  Rate Limiter Dynamic2/1 -> Out2/1, Out1/1

== system PneumaticsSystem/PneumaticsPerVehicle/PneumaticsSystem/BogiePneumaticSystems/BrakingSystem/BrakingSystemPerBogie/BrakeControlUnit/BECUFaultToTCMS/If Action Subsystem1 ==
  In1 : Inport
  Action Port : ActionPort  ActionPortLabel=else
  Gain : Gain
  Out1 : Outport
  wires:
  In1/1 -> Gain/1
  Gain/1 -> Out1/1

== system PneumaticsSystem/PneumaticsPerVehicle/PneumaticsSystem/BogiePneumaticSystems/BrakingSystem/BrakingSystemPerBogie/BrakeControlUnit/BECUFaultToTCMS/If Action Subsystem4 ==
  In1 : Inport
  Action Port : ActionPort  InitializeStates=reset  ActionPortLabel=elseif(u1 < 40)
  Out1 : Outport  OutputWhenDisabled=reset  InitialOutput=0
  wires:
  In1/1 -> Out1/1

== system PneumaticsSystem/PneumaticsPerVehicle/PneumaticsSystem/BogiePneumaticSystems/BrakingSystem/BrakingSystemPerBogie/BrakeControlUnit/BECUFaultToTCMS/If Action Subsystem5 ==
  In1 : Inport
  Action Port : ActionPort  InitializeStates=reset  ActionPortLabel=if(u1 > 80)
  Out1 : Outport  OutputWhenDisabled=reset  InitialOutput=0
  wires:
  In1/1 -> Out1/1

== system PneumaticsSystem/PneumaticsPerVehicle/PneumaticsSystem/BogiePneumaticSystems/BrakingSystem/BrakingSystemPerBogie/BrakeControlUnit/BECUFaultToTCMS/If Action Subsystem6 ==
  In1 : Inport
  Action Port : ActionPort  InitializeStates=reset  ActionPortLabel=elseif( (u1 > 40)&(u1 < 80))
  Out1 : Outport  OutputWhenDisabled=reset  InitialOutput=0
  wires:
  In1/1 -> Out1/1

== system PneumaticsSystem/PneumaticsPerVehicle/PneumaticsSystem/BogiePneumaticSystems/BrakingSystem/BrakingSystemPerBogie/BrakeCylinderSystemPerAxle/AxleBrakeCylinder/FlowCalc ==
  note: Need to Isolate on pressure difference
      | within deadband to stop oscillations.
      | Deadband on Valve is for BSR and BC pressure.
  BSRPressure : Inport
  ControlPressure : Inport  Port=2
  BCPressure : Inport  Port=3
  BCIsolCock : Inport  Port=4
  Abs : Abs
  Add : Sum  Inputs=+--
  BC Charge : PneumaticLib/SS One Way Valve Variable  p_deadband=1000
      settings: SourceProductName=Train Library
  BC Isolate : PneumaticLib/SS One Way Valve  d=0.015  p_deadband=1000
      settings: SourceProductName=Train Library
  BC Vent : PneumaticLib/SS One Way Valve Variable  p_deadband=500
      settings: SourceProductName=Train Library
  Charge Choke : PneumaticLib/Variable Orifice  FullDiam=0.0032  DiffGain=0.0001
      settings: SourceProductName=Train Library
  Compare To Constant : simulink/Logic and Bit Operations/Compare To Constant  relop=<=  const=1000  OutDataTypeStr=boolean
  Constant : Constant  Value=PAtm
  Logical Operator1 : Logic  Operator=NOT  AllPortsSameDT=off  OutDataTypeStr=boolean
  Logical Operator2 : Logic  Operator=OR  AllPortsSameDT=off  OutDataTypeStr=boolean
  Release Choke : PneumaticLib/Variable Orifice  FullDiam=0.008  DiffGain=0.0002
      settings: SourceProductName=Train Library
  Subtract : Sum  Inputs=+-
  Terminator : Terminator
  Terminator1 : Terminator
  Terminator2 : Terminator
  Flow : Outport
  BSRtoBCFlow : Outport  Port=2
  wires:
  ControlPressure/1 -> Charge Choke/1, Release Choke/2, Subtract/2
  BC Charge/1 -> BSRtoBCFlow/1, Add/1
  BCPressure/1 -> BC Isolate/1, Subtract/1, Release Choke/1, BC Vent/1, Charge Choke/2, BC Charge/2
  Add/1 -> Flow/1
  BC Charge/2 -> Terminator/1
  BC Vent/2 -> Terminator1/1
  BC Vent/1 -> Add/2
  BSRPressure/1 -> BC Charge/1
  Charge Choke/1 -> BC Charge/3
  Release Choke/1 -> BC Vent/3
  Constant/1 -> BC Vent/2, BC Isolate/2
  BCIsolCock/1 -> BC Isolate/3, Logical Operator1/1
  BC Isolate/1 -> Add/3
  BC Isolate/2 -> Terminator2/1
  Subtract/1 -> Abs/1
  Abs/1 -> Compare To Constant/1
  Compare To Constant/1 -> Logical Operator2/1
  Logical Operator1/1 -> Logical Operator2/2
  Logical Operator2/1 -> BC Vent/4, BC Charge/4

== matlab function PneumaticsSystem/MRPipeState/UpDnSel ==
  data: u input; yUp output; yDn output
function [yUp, yDn] = UpDnSel(u)
    yUp = [0;u(1:length(u)-1)];
    yDn = [u(2:length(u));0];
end

== matlab function PneumaticsSystem/MRPipeState/PipeConnections ==
  data: frontCock input; rearCock input; frontState output; rearState output; frontCoupled input; rearCoupled input
function [frontState , rearState] = PipeConnections(frontCock,rearCock,frontCoupled,rearCoupled)
%#codegen
    
    CONNECTED = 1.0;
    CONNECTED_ATM = 2.0;
    
    rearCockUp = [0;rearCock(1:length(rearCock)-1)];
    frontCockDown = [frontCock(2:length(frontCock));0];

    frontState = zeros(length(frontCock), 1);
    rearState = zeros(length(rearCock), 1);
    for i=1:length(frontCock)
      if frontCock(i)== 1 && frontCoupled(i) == 1
        if rearCockUp(i) == 1
          frontState(i) = CONNECTED;
        else
          frontState(i) = CONNECTED_ATM;
        end
      end
      if rearCock(i) == 1 && rearCoupled(i) == 1
        if frontCockDown(i) == 1
          rearState(i) = CONNECTED;
        else
          rearState(i) = CONNECTED_ATM;
        end
      end
    end
end
